simulink model "min_max_proj_axis"  (R2018a)
settings: Solver=VariableStepAuto  StartTime=0.0  StopTime=10.0  RelTol=1e-3
settings Model: Creator=Rafael  LastModifiedBy=Rafael
settings DataIOCC: SaveOutput=off  SaveTime=off

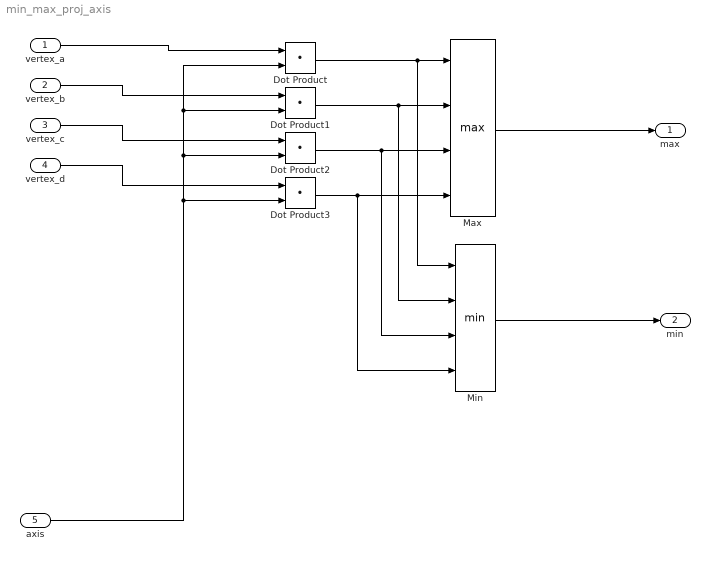
== system min_max_proj_axis ==
  vertex_a : Inport  OutDataTypeStr=double  PortDimensions=2  SampleTime=0
  vertex_b : Inport  Port=2  OutDataTypeStr=double  PortDimensions=2  SampleTime=0
  vertex_c : Inport  Port=3  OutDataTypeStr=double  PortDimensions=2  SampleTime=0
  vertex_d : Inport  Port=4  OutDataTypeStr=double  PortDimensions=2  SampleTime=0
  "axis " : Inport  Port=5  OutDataTypeStr=double  PortDimensions=2  SampleTime=0
  Dot Product{,1..3} (4 alike) : DotProduct  InputSameDT=on  OutDataTypeStr=Inherit: Inherit via internal rule
  Max : MinMax  Function=max  Inputs=4
  Min : MinMax  Inputs=4
  max : Outport  OutDataTypeStr=double  PortDimensions=1  SampleTime=0
  min : Outport  Port=2  OutDataTypeStr=double  PortDimensions=1  SampleTime=0
  wires:
  vertex_c/1 -> Dot Product2/1
  "axis "/1 -> Dot Product/2, Dot Product1/2, Dot Product2/2, Dot Product3/2
  Max/1 -> max/1
  Dot Product2/1 -> Max/3, Min/3
  vertex_d/1 -> Dot Product3/1
  Dot Product1/1 -> Max/2, Min/2
  Min/1 -> min/1
  Dot Product3/1 -> Max/4, Min/4
  Dot Product/1 -> Max/1, Min/1
  vertex_a/1 -> Dot Product/1
  vertex_b/1 -> Dot Product1/1
